simulink subsystem "BMS"  (R2023b)
settings: Solver=VariableStepAuto  StartTime=0.0  StopTime=10.0  RelTol=1e-3
undefined symbols (not defined in the file): C1_LUT, C2_LUT, DiscIntNeverNeededParam, OCV_LUT, R0_LUT, R1_LUT, R2_LUT, rCellCapacity, SoC_LUT, tSimBattMgt
libraries: simulink x3
settings Model: DataDictionary=BatteryManagement_data.sldd  EnableAccessToBaseWorkspace=off  Creator=Elio  LastModifiedBy=Elio

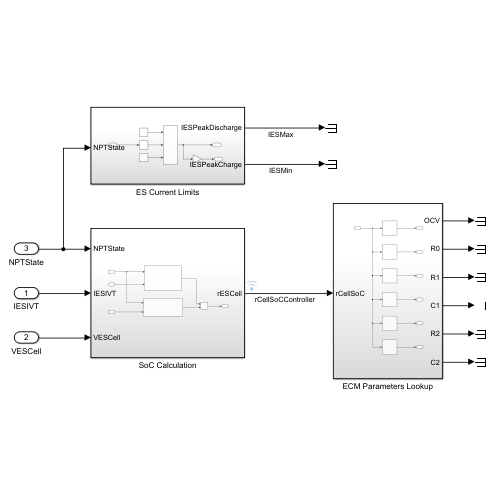
[thumbnail: Simulink's stored preview of the top-level diagram]
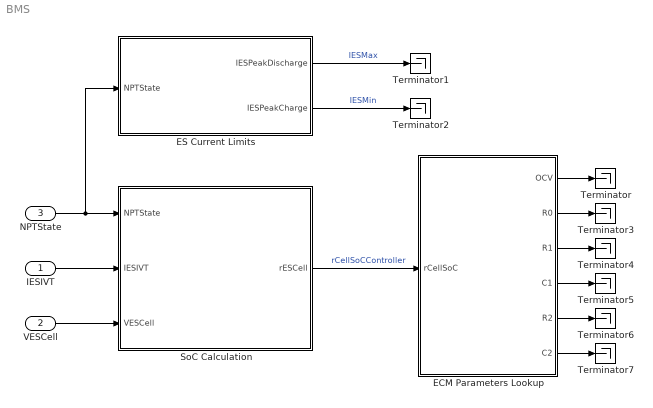
== system BMS ==
  IESIVT : Inport
  VESCell : Inport  Port=2
  NPTState : Inport  Port=3
  ECM Parameters Lookup : Subsystem
  ES Current Limits : Subsystem
  SoC Calculation : Subsystem
  Terminator{,1..7} (8 alike) : Terminator
  wires:
  ECM Parameters Lookup/4(C1) -> Terminator5/1
  ECM Parameters Lookup/5(R2) -> Terminator6/1
  ECM Parameters Lookup/3(R1) -> Terminator4/1
  SoC Calculation/1(rESCell) -> ECM Parameters Lookup/1(rCellSoC)  "rCellSoCController"
  ECM Parameters Lookup/2(R0) -> Terminator3/1
  ECM Parameters Lookup/1(OCV) -> Terminator/1
  IESIVT/1 -> SoC Calculation/2(IESIVT)
  VESCell/1 -> SoC Calculation/3(VESCell)
  NPTState/1 -> ES Current Limits/1(NPTState), SoC Calculation/1(NPTState)
  ES Current Limits/1(IESPeakDischarge) -> Terminator1/1  "IESMax"
  ECM Parameters Lookup/6(C2) -> Terminator7/1
  ES Current Limits/2(IESPeakCharge) -> Terminator2/1  "IESMin"

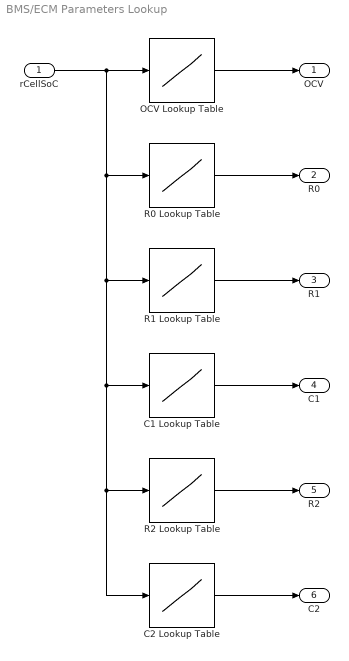
== system BMS/ECM Parameters Lookup ==
  rCellSoC : Inport
  C1 Lookup Table : Lookup_n-D  NumberOfTableDimensions=1  LookupTableObject=''  BreakpointsForDimension1=SoC_LUT  BreakpointsForDimension1FirstPoint=10  BreakpointsForDimension2FirstPoint=10  BreakpointsForDimension1Spacing=12  BreakpointsForDimension2Spacing=12  IndexSearchMethod=Evenly spaced points  Table=C1_LUT  DiagnosticForOutOfRangeInput=Error  InternalRulePriority=Speed  RndMeth=Simplest
  C2 Lookup Table : Lookup_n-D  NumberOfTableDimensions=1  LookupTableObject=''  BreakpointsForDimension1=SoC_LUT  BreakpointsForDimension1FirstPoint=10  BreakpointsForDimension2FirstPoint=10  BreakpointsForDimension1Spacing=12  BreakpointsForDimension2Spacing=12  IndexSearchMethod=Evenly spaced points  Table=C2_LUT  DiagnosticForOutOfRangeInput=Error  InternalRulePriority=Speed  RndMeth=Simplest
  OCV Lookup Table : Lookup_n-D  NumberOfTableDimensions=1  LookupTableObject=''  BreakpointsForDimension1=SoC_LUT  BreakpointsForDimension1FirstPoint=10  BreakpointsForDimension2FirstPoint=10  BreakpointsForDimension1Spacing=12  BreakpointsForDimension2Spacing=12  Table=OCV_LUT  DiagnosticForOutOfRangeInput=Error  InternalRulePriority=Speed  RndMeth=Simplest
  R0 Lookup Table : Lookup_n-D  NumberOfTableDimensions=1  LookupTableObject=''  BreakpointsForDimension1=SoC_LUT  BreakpointsForDimension1FirstPoint=10  BreakpointsForDimension2FirstPoint=10  BreakpointsForDimension1Spacing=12  BreakpointsForDimension2Spacing=12  IndexSearchMethod=Evenly spaced points  Table=R0_LUT  DiagnosticForOutOfRangeInput=Error  InternalRulePriority=Speed  RndMeth=Simplest
  R1 Lookup Table : Lookup_n-D  NumberOfTableDimensions=1  LookupTableObject=''  BreakpointsForDimension1=SoC_LUT  BreakpointsForDimension1FirstPoint=10  BreakpointsForDimension2FirstPoint=10  BreakpointsForDimension1Spacing=12  BreakpointsForDimension2Spacing=12  IndexSearchMethod=Evenly spaced points  Table=R1_LUT  DiagnosticForOutOfRangeInput=Error  InternalRulePriority=Speed  RndMeth=Simplest
  R2 Lookup Table : Lookup_n-D  NumberOfTableDimensions=1  LookupTableObject=''  BreakpointsForDimension1=SoC_LUT  BreakpointsForDimension1FirstPoint=10  BreakpointsForDimension2FirstPoint=10  BreakpointsForDimension1Spacing=12  BreakpointsForDimension2Spacing=12  IndexSearchMethod=Evenly spaced points  Table=R2_LUT  DiagnosticForOutOfRangeInput=Error  InternalRulePriority=Speed  RndMeth=Simplest
  OCV : Outport
  R0 : Outport  Port=2
  R1 : Outport  Port=3
  C1 : Outport  Port=4
  R2 : Outport  Port=5
  C2 : Outport  Port=6
  wires:
  rCellSoC/1 -> R1 Lookup Table/1, C2 Lookup Table/1, R2 Lookup Table/1, C1 Lookup Table/1, R0 Lookup Table/1, OCV Lookup Table/1
  OCV Lookup Table/1 -> OCV/1
  R0 Lookup Table/1 -> R0/1
  R1 Lookup Table/1 -> R1/1
  C1 Lookup Table/1 -> C1/1
  R2 Lookup Table/1 -> R2/1
  C2 Lookup Table/1 -> C2/1

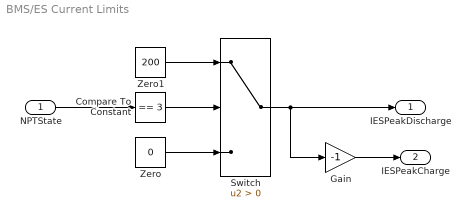
== system BMS/ES Current Limits ==
  NPTState : Inport
  Compare To Constant : simulink/Logic and Bit Operations/Compare To Constant  relop===  const=3  OutDataTypeStr=boolean
  Gain : Gain  Gain=-1
  Switch : Switch  Criteria=u2 > Threshold  SaturateOnIntegerOverflow=off  InputSameDT=off
  Zero : Constant  Value=0  OutDataTypeStr=Inherit: Inherit via back propagation  SampleTime=tSimBattMgt
  Zero1 : Constant  Value=200  OutDataTypeStr=Inherit: Inherit via back propagation  SampleTime=tSimBattMgt
  IESPeakDischarge : Outport
  IESPeakCharge : Outport  Port=2
  wires:
  Compare To Constant/1 -> Switch/2
  Zero/1 -> Switch/3
  Switch/1 -> Gain/1, IESPeakDischarge/1
  Zero1/1 -> Switch/1
  NPTState/1 -> Compare To Constant/1
  Gain/1 -> IESPeakCharge/1

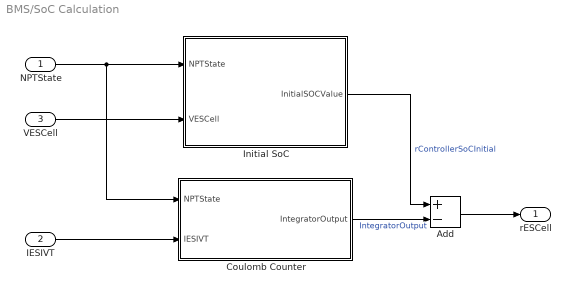
== system BMS/SoC Calculation ==
  NPTState : Inport
  IESIVT : Inport  Port=2
  VESCell : Inport  Port=3
  Add : Sum  Inputs=+-
  Coulomb Counter : Subsystem  TreatAsAtomicUnit=on
  Initial SoC : Subsystem
  rESCell : Outport
  wires:
  Add/1 -> rESCell/1
  Coulomb Counter/1(IntegratorOutput) -> Add/2  "IntegratorOutput"
  IESIVT/1 -> Coulomb Counter/2(IESIVT)
  Initial SoC/1(InitialSOCValue) -> Add/1  "rControllerSoCInitial"
  VESCell/1 -> Initial SoC/2(VESCell)
  NPTState/1 -> Coulomb Counter/1(NPTState), Initial SoC/1(NPTState)

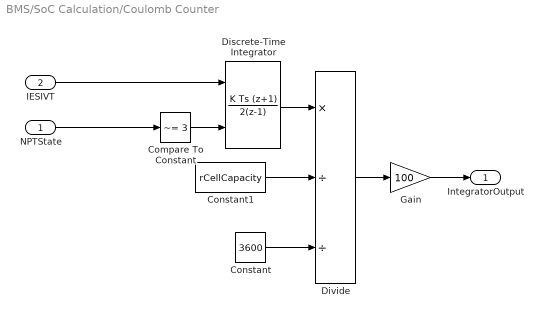
== system BMS/SoC Calculation/Coulomb Counter ==
  NPTState : Inport
  IESIVT : Inport  Port=2
  Compare To Constant : simulink/Logic and Bit Operations/Compare To Constant  relop=~=  const=3  OutDataTypeStr=boolean
  Constant : Constant  Value=3600  SampleTime=tSimBattMgt
  Constant1 : Constant  Value=rCellCapacity  SampleTime=tSimBattMgt
  Discrete-Time Integrator : DiscreteIntegrator  IntegratorMethod=Integration: Trapezoidal  ExternalReset=rising  SampleTime=-1  ICPrevOutput=DiscIntNeverNeededParam  ICPrevScaledInput=DiscIntNeverNeededParam
  Divide : Product  Inputs=*//
  Gain : Gain  Gain=100
  IntegratorOutput : Outport
  wires:
  Divide/1 -> Gain/1
  Constant1/1 -> Divide/2
  Discrete-Time Integrator/1 -> Divide/1
  Constant/1 -> Divide/3
  IESIVT/1 -> Discrete-Time Integrator/1
  Gain/1 -> IntegratorOutput/1
  Compare To Constant/1 -> Discrete-Time Integrator/2
  NPTState/1 -> Compare To Constant/1

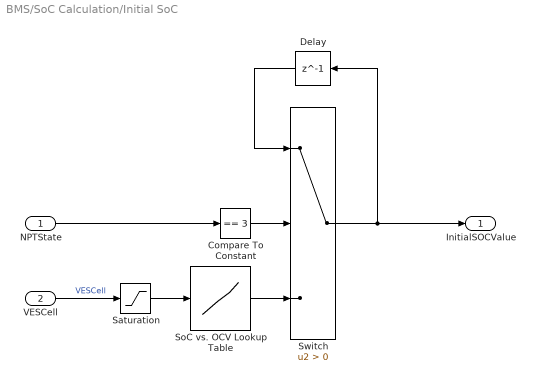
== system BMS/SoC Calculation/Initial SoC ==
  NPTState : Inport
  VESCell : Inport  Port=2
  Compare To Constant : simulink/Logic and Bit Operations/Compare To Constant  relop===  const=3  OutDataTypeStr=boolean
  Delay : Delay  DelayLength=1
  Saturation : Saturate  UpperLimit=4.182  LowerLimit=2.8
  SoC vs. OCV Lookup Table : Lookup_n-D  NumberOfTableDimensions=1  LookupTableObject=''  BreakpointsForDimension1=OCV_LUT  BreakpointsForDimension1FirstPoint=10  BreakpointsForDimension2FirstPoint=10  BreakpointsForDimension1Spacing=12  BreakpointsForDimension2Spacing=12  Table=SoC_LUT  DiagnosticForOutOfRangeInput=Error  InternalRulePriority=Speed  RndMeth=Simplest
  Switch : Switch  Criteria=u2 > Threshold  SaturateOnIntegerOverflow=off  InputSameDT=off
  InitialSOCValue : Outport
  wires:
  Compare To Constant/1 -> Switch/2
  Switch/1 -> Delay/1, InitialSOCValue/1
  SoC vs. OCV Lookup Table/1 -> Switch/3
  NPTState/1 -> Compare To Constant/1
  VESCell/1 -> Saturation/1  "VESCell"
  Delay/1 -> Switch/1
  Saturation/1 -> SoC vs. OCV Lookup Table/1
